simulink model "AnodeSubsystem_without_stack_Simplified"  (R2023a)
settings: Solver=VariableStepAuto  StartTime=0.0  StopTime=80  RelTol=1e-3
values from neighbouring files (symbols this model uses):
  anode_tube_D = 0.01    [Initialization_Anode.m]
  D = 0.01    [Initialization_Anode.m]
  densityHydrogen = 0.0899    [Initialization_Anode.m]
  Kv_VL6112 = 0.80    (= 0.8)    [Initialization_Anode.m]
  N2_T = [-56.55, -50:10:-10, -5:1:5, 10:10:350]    [Initialization_Anode.m]
  p_range = 0.005    [Initialization_Anode.m]
  r_max = 0.2    [Initialization_Anode.m]
  r_min = 1e-4    (= 0.0001)    [Initialization_Anode.m]
  responseTimeValve = 0.013    [Initialization_Anode.m]
libraries: fl_lib x64, nesl_utility x40, SimscapeFluids_lib x1
(part 2 of 2)

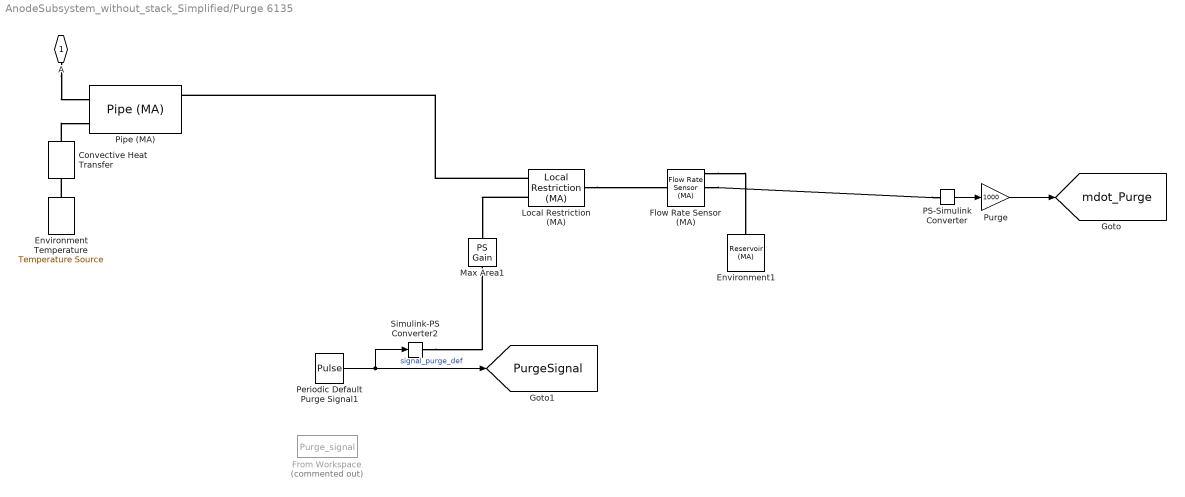
== system AnodeSubsystem_without_stack_Simplified/Purge 6135 ==
  Convective Heat Transfer : fl_lib/Thermal/Thermal Elements/Convective Heat Transfer  thermal_type=foundation.enum.constant_variable.constant  area=pi*anode_tube_D*1 m^2  heat_tr_coeff=20 W/(m^2 * K)  min_heat_tr_coeff=1e-3 W/(K*m^2)  T_specify=off  T_priority=None  T=0 K  T_nominal_specify=off  T_nominal_unit=K  T_nominal_value=1  Q_specify=off  Q_priority=None  Q=0 W  Q_nominal_specify=off  Q_nominal_unit=W  Q_nominal_value=1
  Environment Temperature : fl_lib/Thermal/Thermal Sources/Temperature Source  temperature=env_T degC
  Environment1 : fl_lib/Moist Air/Elements/Reservoir (MA)  pressure_spec=foundation.enum.pressure_spec.atmospheric  reservoir_pressure=0.101325 MPa  temperature_spec=foundation.enum.temperature_spec.atmospheric  reservoir_temperature=293.15 K  moisture_spec=foundation.enum.moistureSpec.RelativeHumidity  reservoir_RH=0.5  reservoir_x_w=0.01  reservoir_y_w=0.01  reservoir_HR=0.01  reservoir_Tw=287 K  trace_gas_spec=foundation.enum.trace_gas_spec.mass_fraction  reservoir_x_g=0.001  reservoir_y_g=0.001  RH_ws=1  area_A=0.01 m^2
  Flow Rate Sensor (MA) : fl_lib/Moist Air/Sensors/Flow Rate Sensor (MA)  mass_flow_measure=true  volumetric_flow_measure=false  volumetric_flow_conditions=foundation.enum.volumetric_flow_conditions.actual  p_std=0.101325 MPa  T_std=20 degC  RH_std=0.65  energy_flow_measure=true  vapor_flow_measure=false  gas_flow_measure=false
      settings: InternalSimscapePortConfiguration="{\"Bottom\":[{\"id\":\"PHI\",\"label\":\"φ\",\"type\":\"output\"}],\"Left\":[{\"id\":\"A\",\"label\":\"A\",\"type\":\"foundation.moist_air.moist_air\"}],\"Right\":[{\"id\":\"B\",\"label\":\"B\",\"type\":\"foundation.moist_air.moist_air\"},{\"id\":\"M\",\"label\":\"M\",\"type\":\"output\"}],\"Top\":[]}"
  From Workspace : FromWorkspace  Commented=on  VariableName=Purge_signal
  Local Restriction (MA) : fl_lib/Moist Air/Elements/Local Restriction (MA)  restriction_type=foundation.enum.restriction_type.variable  restriction_area=0.005 m^2  min_area=0.00001e-6 m^2  max_area=3.2e-6 m^2  area=0.00358 m^2  Cd=0.80  B_lam=0.999
      settings: LogSimulationData=on
  Max Area1 : fl_lib/Physical Signals/Functions/PS Gain  gain=3.2e-6 m^2
  PS-Simulink Converter : nesl_utility/PS-Simulink Converter  PhysicalDomain=network_engine_domain  SubClassName=ps_output  LeftPortType=input  RightPortType=output  PseudoPeriodic=off  Frequencies=[]  VectorFormat=inherit  Unit=inherit  AffineConversion=off
  Periodic Default Purge Signal1 : DiscretePulseGenerator  PulseType=Time based  Period=3  PulseWidth=5
  Pipe (MA) : fl_lib/Moist Air/Elements/Pipe (MA)  length=1 m  area=pi*anode_tube_D^2/4 m^2  Dh=anode_tube_D m  length_add=0.1 m  roughness=15e-6 m  Re_lam=2000  Re_tur=4000  shape_factor=64  Nu_lam=3.66  wall_condensation=simscape.enum.onoff.off  RH_ws=1  time_constant=1e-3 s  moisture_trace_gas_source=foundation.enum.moisture_trace_gas_source.none  moisture_source_spec=foundation.enum.moisture_source_spec.vapor  moisture_mass_flow=0 kg/s  moisture_temperature_spec=foundation.enum.temperature_spec.atmospheric  moisture_temperature=293.15 K  trace_gas_mass_flow=0 kg/s  trace_gas_temperature_spec=foundation.enum.temperature_spec.atmospheric  trace_gas_temperature=293.15 K  p_I_specify=on  p_I_priority=High  p_I=env_p MPa  p_I_nominal_specify=off  p_I_nominal_unit=MPa  p_I_nominal_value=1  T_I_specify=on  T_I_priority=High  T_I=env_T degC  T_I_nominal_specify=off  T_I_nominal_unit=K  T_I_nominal_value=1  RH_I_specify=off  RH_I_priority=High  RH_I=0  RH_I_nominal_specify=off  RH_I_nominal_unit=1  RH_I_nominal_value=1  x_w_I_specify=off  x_w_I_priority=None  x_w_I=0  x_w_I_nominal_specify=off  x_w_I_nominal_unit=1  x_w_I_nominal_value=1  y_w_I_specify=off  y_w_I_priority=None  y_w_I=0  y_w_I_nominal_specify=off  y_w_I_nominal_unit=1  y_w_I_nominal_value=1  HR_I_specify=off  HR_I_priority=None  HR_I=0  HR_I_nominal_specify=off  HR_I_nominal_unit=1  HR_I_nominal_value=1  x_g_I_specify=on  x_g_I_priority=None  x_g_I=0  x_g_I_nominal_specify=off  x_g_I_nominal_unit=1  x_g_I_nominal_value=1  y_g_I_specify=on  y_g_I_priority=High  y_g_I=tank_yH2  y_g_I_nominal_specify=off  y_g_I_nominal_unit=1  y_g_I_nominal_value=1
  Purge : Gain  Gain=1000
  Simulink-PS Converter2 : nesl_utility/Simulink-PS Converter  PhysicalDomain=network_engine_domain  SubClassName=ps_input  LeftPortType=input  RightPortType=output  PseudoPeriodic=off  Frequencies=[]  NoiseDistribution=none  NoiseParameters=[]  Unit=1  AffineConversion=off  FilteringAndDerivatives=provide  SimscapeFilterOrder=1  InputFilterTimeConstant=0.001  UdotUserProvided=0
  A : PMIOPort  Side=Left
  tag scope: PurgeSignal=global, mdot_Purge=global
  wires:
  PS-Simulink Converter/1 -> Purge/1
  Purge/1 -> [mdot_Purge]
  Periodic Default Purge Signal1/1 -> [PurgeSignal], Simulink-PS Converter2/1  "signal_purge_def"
  connections:
  Environment Temperature/LConn1 -- Convective Heat Transfer/RConn1
  Convective Heat Transfer/LConn1 -- Pipe (MA)/LConn2
  A/RConn1 -- Pipe (MA)/LConn1
  Local Restriction (MA)/LConn2 -- Max Area1/RConn1
  Simulink-PS Converter2/RConn1 -- Max Area1/LConn1
  Local Restriction (MA)/LConn1 -- Pipe (MA)/RConn1
  Local Restriction (MA)/RConn1 -- Flow Rate Sensor (MA)/LConn1
  Flow Rate Sensor (MA)/RConn1 -- Environment1/LConn1
  Flow Rate Sensor (MA)/RConn2 -- PS-Simulink Converter/LConn1

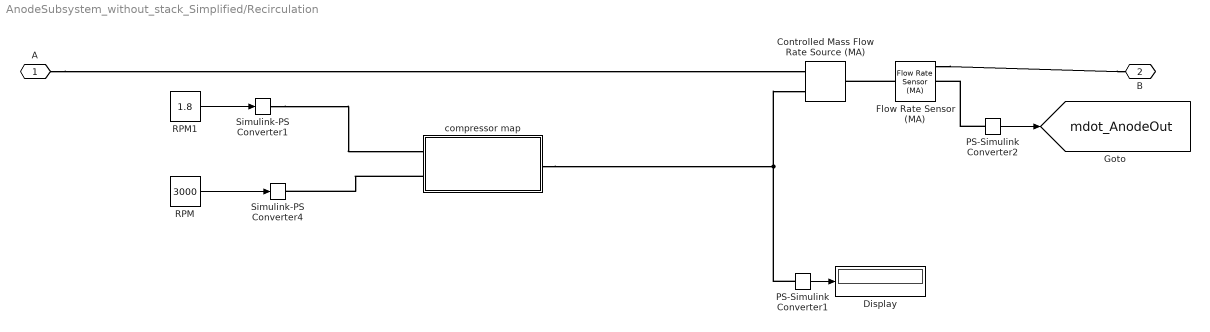
== system AnodeSubsystem_without_stack_Simplified/Recirculation ==
  Controlled Mass Flow Rate Source (MA) : fl_lib/Moist Air/Sources/Controlled Mass Flow Rate Source (MA)  power_spec=foundation.enum.power_spec.isentropic  area_A=pi*anode_tube_D^2/4 m^2  area_B=pi*anode_tube_D^2/4 m^2
      settings: InternalSimscapePortConfiguration="{\"Bottom\":[],\"Left\":[{\"id\":\"A\",\"label\":\"A\",\"type\":\"foundation.moist_air.moist_air\"},{\"id\":\"M\",\"label\":\"M\",\"type\":\"input\"}],\"Right\":[{\"id\":\"B\",\"label\":\"B\",\"type\":\"foundation.moist_air.moist_air\"}],\"Top\":[]}"
  Display : Display
  Flow Rate Sensor (MA) : fl_lib/Moist Air/Sensors/Flow Rate Sensor (MA)  mass_flow_measure=true  volumetric_flow_measure=false  volumetric_flow_conditions=foundation.enum.volumetric_flow_conditions.actual  p_std=0.101325 MPa  T_std=20 degC  RH_std=0.65  energy_flow_measure=true  vapor_flow_measure=false  gas_flow_measure=false
      settings: InternalSimscapePortConfiguration="{\"Bottom\":[{\"id\":\"PHI\",\"label\":\"φ\",\"type\":\"output\"}],\"Left\":[{\"id\":\"A\",\"label\":\"A\",\"type\":\"foundation.moist_air.moist_air\"}],\"Right\":[{\"id\":\"B\",\"label\":\"B\",\"type\":\"foundation.moist_air.moist_air\"},{\"id\":\"M\",\"label\":\"M\",\"type\":\"output\"}],\"Top\":[]}"
  PS-Simulink Converter1 : nesl_utility/PS-Simulink Converter  PhysicalDomain=network_engine_domain  SubClassName=ps_output  LeftPortType=input  RightPortType=output  PseudoPeriodic=off  Frequencies=[]  VectorFormat=inherit  Unit=inherit  AffineConversion=off
  PS-Simulink Converter2 : nesl_utility/PS-Simulink Converter  PhysicalDomain=network_engine_domain  SubClassName=ps_output  LeftPortType=input  RightPortType=output  PseudoPeriodic=off  Frequencies=[]  VectorFormat=inherit  Unit=inherit  AffineConversion=off
  RPM : Constant  Value=3000
  RPM1 : Constant  Value=1.8
  Simulink-PS Converter1 : nesl_utility/Simulink-PS Converter  PhysicalDomain=network_engine_domain  SubClassName=ps_input  LeftPortType=input  RightPortType=output  PseudoPeriodic=off  Frequencies=[]  NoiseDistribution=none  NoiseParameters=[]  Unit=1  AffineConversion=off  FilteringAndDerivatives=provide  SimscapeFilterOrder=1  InputFilterTimeConstant=0.001  UdotUserProvided=0
  Simulink-PS Converter4 : nesl_utility/Simulink-PS Converter  PhysicalDomain=network_engine_domain  SubClassName=ps_input  LeftPortType=input  RightPortType=output  PseudoPeriodic=off  Frequencies=[]  NoiseDistribution=none  NoiseParameters=[]  Unit=1  AffineConversion=off  FilteringAndDerivatives=provide  SimscapeFilterOrder=1  InputFilterTimeConstant=0.001  UdotUserProvided=0
  compressor map : Subsystem
  A : PMIOPort  Side=Left
  B : PMIOPort  Port=2  Side=Right
  tag scope: mdot_AnodeOut=global
  wires:
  RPM/1 -> Simulink-PS Converter4/1
  PS-Simulink Converter1/1 -> Display/1
  PS-Simulink Converter2/1 -> [mdot_AnodeOut]
  RPM1/1 -> Simulink-PS Converter1/1
  connections:
  A/RConn1 -- Controlled Mass Flow Rate Source (MA)/LConn1
  compressor map/LConn2 -- Simulink-PS Converter4/RConn1
  compressor map/RConn1 -- PS-Simulink Converter1/LConn1 -- Controlled Mass Flow Rate Source (MA)/LConn2
  Flow Rate Sensor (MA)/LConn1 -- Controlled Mass Flow Rate Source (MA)/RConn1
  Flow Rate Sensor (MA)/RConn1 -- B/RConn1
  PS-Simulink Converter2/LConn1 -- Flow Rate Sensor (MA)/RConn2
  Simulink-PS Converter1/RConn1 -- compressor map/LConn1

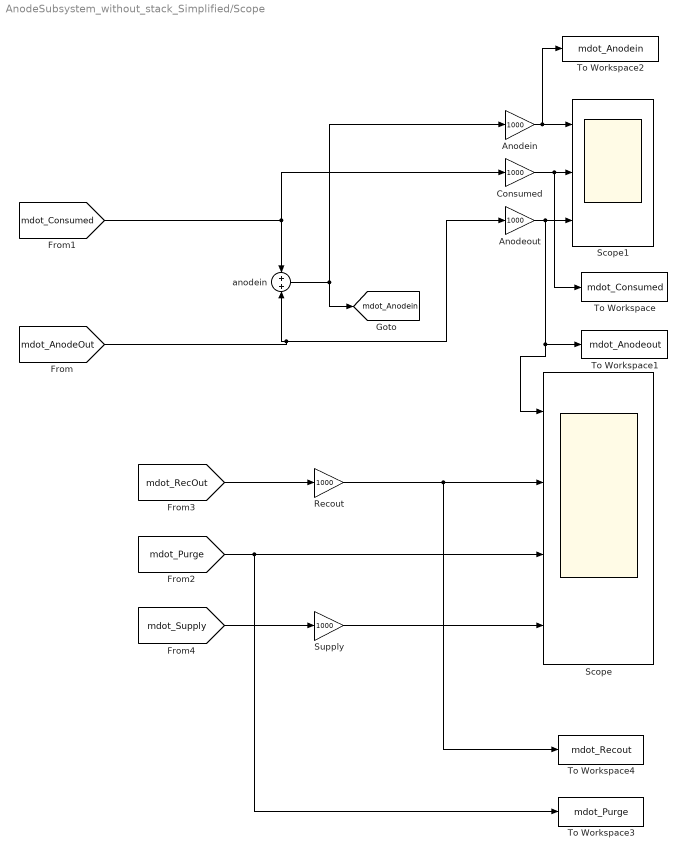
== system AnodeSubsystem_without_stack_Simplified/Scope ==
  Anodein : Gain  Gain=1000
  Anodeout : Gain  Gain=1000
  Consumed : Gain  Gain=1000
  Recout : Gain  Gain=1000
  Scope : Scope  NumInputPorts=4
  Scope1 : Scope  NumInputPorts=3
  Supply : Gain  Gain=1000
  To Workspace : ToWorkspace  VariableName=mdot_Consumed  SaveFormat=Structure With Time  SampleTime=-1
  To Workspace1 : ToWorkspace  VariableName=mdot_Anodeout  SaveFormat=Structure With Time  SampleTime=-1
  To Workspace2 : ToWorkspace  VariableName=mdot_Anodein  SaveFormat=Structure With Time  SampleTime=-1
  To Workspace3 : ToWorkspace  VariableName=mdot_Purge  SaveFormat=Structure With Time  SampleTime=-1
  To Workspace4 : ToWorkspace  VariableName=mdot_Recout  SaveFormat=Structure With Time  SampleTime=-1
  anodein : Sum
  tag scope: mdot_Anodein=global
  wires:
  [mdot_Consumed] -> anodein/1, Consumed/1
  [mdot_AnodeOut] -> Anodeout/1, anodein/2
  Anodein/1 -> To Workspace2/1, Scope1/1
  Anodeout/1 -> Scope/1, To Workspace1/1, Scope1/3
  Consumed/1 -> To Workspace/1, Scope1/2
  [mdot_Purge] -> To Workspace3/1, Scope/3
  anodein/1 -> [mdot_Anodein], Anodein/1
  Recout/1 -> To Workspace4/1, Scope/2
  [mdot_RecOut] -> Recout/1
  [mdot_Supply] -> Supply/1
  Supply/1 -> Scope/4

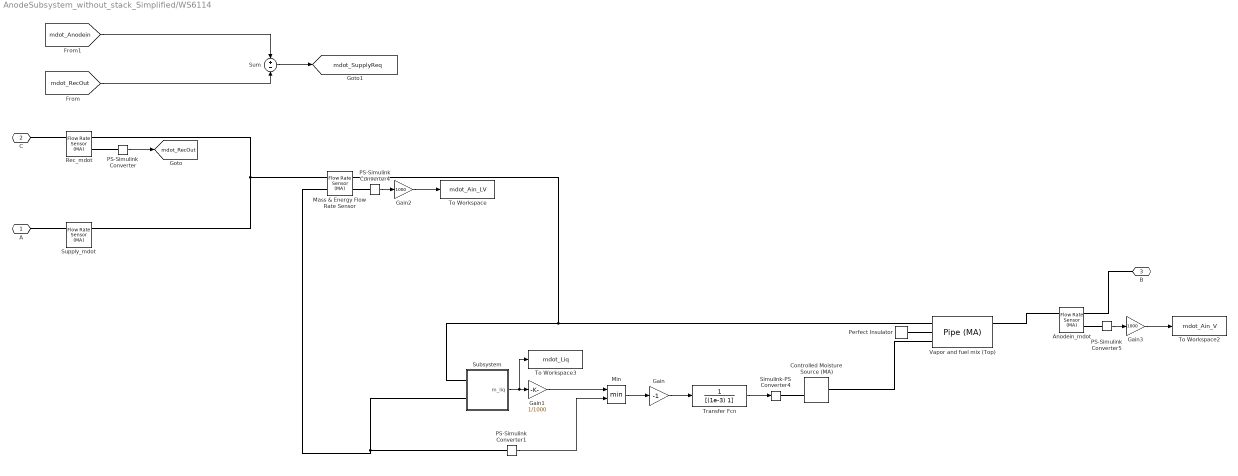
== system AnodeSubsystem_without_stack_Simplified/WS6114 ==
  Anodein_mdot : fl_lib/Moist Air/Sensors/Flow Rate Sensor (MA)  mass_flow_measure=true  volumetric_flow_measure=false  volumetric_flow_conditions=foundation.enum.volumetric_flow_conditions.actual  p_std=0.101325 MPa  T_std=20 degC  RH_std=0.65  energy_flow_measure=false  vapor_flow_measure=true  gas_flow_measure=false
      settings: InternalSimscapePortConfiguration="{\"Bottom\":[],\"Left\":[{\"id\":\"A\",\"label\":\"A\",\"type\":\"foundation.moist_air.moist_air\"},{\"id\":\"Mw\",\"label\":\"Mw\",\"type\":\"output\"}],\"Right\":[{\"id\":\"B\",\"label\":\"B\",\"type\":\"foundation.moist_air.moist_air\"},{\"id\":\"M\",\"label\":\"M\",\"type\":\"output\"}],\"Top\":[]}"
  Controlled Moisture Source (MA) : fl_lib/Moist Air/Sources/Moisture & Trace Gas Sources/Controlled Moisture Source (MA)  moisture_source_spec=foundation.enum.moisture_source_spec.liquid  Phi_S_specify=off  Phi_S_priority=None  Phi_S=0 kW  Phi_S_nominal_specify=off  Phi_S_nominal_unit=kW  Phi_S_nominal_value=1  mdot_w_S_specify=off  mdot_w_S_priority=None  mdot_w_S=0 kg/s  mdot_w_S_nominal_specify=off  mdot_w_S_nominal_unit=kg/s  mdot_w_S_nominal_value=1
      settings: InternalSimscapePortConfiguration="{\"Bottom\":[],\"Left\":[{\"id\":\"S\",\"label\":\"S\",\"type\":\"foundation.moist_air.moist_air_source\"}],\"Right\":[{\"id\":\"M\",\"label\":\"M\",\"type\":\"input\"},{\"id\":\"T\",\"label\":\"T\",\"type\":\"input\"}],\"Top\":[]}"
  Gain : Gain  Gain=-1
  Gain1 : Gain  Gain=1/1000
  Gain2 : Gain  Gain=1000
  Gain3 : Gain  Gain=1000
  "Mass & Energy Flow Rate Sensor " : fl_lib/Moist Air/Sensors/Flow Rate Sensor (MA)  mass_flow_measure=true  volumetric_flow_measure=false  volumetric_flow_conditions=foundation.enum.volumetric_flow_conditions.actual  p_std=0.101325 MPa  T_std=20 degC  RH_std=0.65  energy_flow_measure=false  vapor_flow_measure=true  gas_flow_measure=false
      settings: InternalSimscapePortConfiguration="{\"Bottom\":[],\"Left\":[{\"id\":\"A\",\"label\":\"A\",\"type\":\"foundation.moist_air.moist_air\"},{\"id\":\"Mw\",\"label\":\"Mw\",\"type\":\"output\"}],\"Right\":[{\"id\":\"B\",\"label\":\"B\",\"type\":\"foundation.moist_air.moist_air\"},{\"id\":\"M\",\"label\":\"M\",\"type\":\"output\"}],\"Top\":[]}"
  Min : MinMax  Inputs=2
  PS-Simulink Converter{,1,4..5} (4 alike) : nesl_utility/PS-Simulink Converter  PhysicalDomain=network_engine_domain  SubClassName=ps_output  LeftPortType=input  RightPortType=output  PseudoPeriodic=off  Frequencies=[]  VectorFormat=inherit  Unit=inherit  AffineConversion=off
  Perfect Insulator : fl_lib/Thermal/Thermal Elements/Perfect Insulator  T_specify=off  T_priority=None  T=0 K  T_nominal_specify=off  T_nominal_unit=K  T_nominal_value=1
  Rec_mdot : fl_lib/Moist Air/Sensors/Flow Rate Sensor (MA)  mass_flow_measure=true  volumetric_flow_measure=false  volumetric_flow_conditions=foundation.enum.volumetric_flow_conditions.actual  p_std=0.101325 MPa  T_std=20 degC  RH_std=0.65  energy_flow_measure=false  vapor_flow_measure=true  gas_flow_measure=false
      settings: InternalSimscapePortConfiguration="{\"Bottom\":[],\"Left\":[{\"id\":\"A\",\"label\":\"A\",\"type\":\"foundation.moist_air.moist_air\"},{\"id\":\"Mw\",\"label\":\"Mw\",\"type\":\"output\"}],\"Right\":[{\"id\":\"B\",\"label\":\"B\",\"type\":\"foundation.moist_air.moist_air\"},{\"id\":\"M\",\"label\":\"M\",\"type\":\"output\"}],\"Top\":[]}"
  Simulink-PS Converter4 : nesl_utility/Simulink-PS Converter  PhysicalDomain=network_engine_domain  SubClassName=ps_input  LeftPortType=input  RightPortType=output  PseudoPeriodic=off  Frequencies=[]  NoiseDistribution=none  NoiseParameters=[]  Unit=1  AffineConversion=off  FilteringAndDerivatives=provide  SimscapeFilterOrder=1  InputFilterTimeConstant=0.001  UdotUserProvided=0
  Subsystem : Subsystem
  Sum : Sum  Inputs=+-
  Supply_mdot : fl_lib/Moist Air/Sensors/Flow Rate Sensor (MA)  mass_flow_measure=true  volumetric_flow_measure=false  volumetric_flow_conditions=foundation.enum.volumetric_flow_conditions.actual  p_std=0.101325 MPa  T_std=20 degC  RH_std=0.65  energy_flow_measure=false  vapor_flow_measure=true  gas_flow_measure=false
      settings: InternalSimscapePortConfiguration="{\"Bottom\":[],\"Left\":[{\"id\":\"A\",\"label\":\"A\",\"type\":\"foundation.moist_air.moist_air\"},{\"id\":\"Mw\",\"label\":\"Mw\",\"type\":\"output\"}],\"Right\":[{\"id\":\"B\",\"label\":\"B\",\"type\":\"foundation.moist_air.moist_air\"},{\"id\":\"M\",\"label\":\"M\",\"type\":\"output\"}],\"Top\":[]}"
  To Workspace : ToWorkspace  VariableName=mdot_Ain_LV  SaveFormat=Structure With Time  SampleTime=-1
  To Workspace2 : ToWorkspace  VariableName=mdot_Ain_V  SaveFormat=Structure With Time  SampleTime=-1
  To Workspace3 : ToWorkspace  VariableName=mdot_Liq  SaveFormat=Structure With Time  SampleTime=-1
  Transfer Fcn : TransferFcn  Denominator=[(1e-3) 1]
  Vapor and fuel mix (Top) : fl_lib/Moist Air/Elements/Pipe (MA)  length=0.25 m  area=pi*0.05^2/4 m^2  Dh=0.05 m  length_add=0.1 m  roughness=15e-6 m  Re_lam=2000  Re_tur=4000  shape_factor=64  Nu_lam=3.66  wall_condensation=simscape.enum.onoff.off  RH_ws=1  time_constant=1e-3 s  moisture_trace_gas_source=foundation.enum.moisture_trace_gas_source.controlled  moisture_source_spec=foundation.enum.moisture_source_spec.vapor  moisture_mass_flow=0 kg/s  moisture_temperature_spec=foundation.enum.temperature_spec.atmospheric  moisture_temperature=293.15 K  trace_gas_mass_flow=0 kg/s  trace_gas_temperature_spec=foundation.enum.temperature_spec.atmospheric  trace_gas_temperature=293.15 K  p_I_specify=on  p_I_priority=High  p_I=env_p MPa  p_I_nominal_specify=off  p_I_nominal_unit=MPa  p_I_nominal_value=1  T_I_specify=on  T_I_priority=High  T_I=env_T degC  T_I_nominal_specify=off  T_I_nominal_unit=K  T_I_nominal_value=1  RH_I_specify=off  RH_I_priority=High  RH_I=0  RH_I_nominal_specify=off  RH_I_nominal_unit=1  RH_I_nominal_value=1  x_w_I_specify=off  x_w_I_priority=None  x_w_I=0  x_w_I_nominal_specify=off  x_w_I_nominal_unit=1  x_w_I_nominal_value=1  y_w_I_specify=off  y_w_I_priority=None  y_w_I=0  y_w_I_nominal_specify=off  y_w_I_nominal_unit=1  y_w_I_nominal_value=1  HR_I_specify=off  HR_I_priority=None  HR_I=0  HR_I_nominal_specify=off  HR_I_nominal_unit=1  HR_I_nominal_value=1  x_g_I_specify=on  x_g_I_priority=None  x_g_I=0  x_g_I_nominal_specify=off  x_g_I_nominal_unit=1  x_g_I_nominal_value=1  y_g_I_specify=on  y_g_I_priority=High  y_g_I=tank_yH2  y_g_I_nominal_specify=off  y_g_I_nominal_unit=1  y_g_I_nominal_value=1
      settings: InternalSimscapePortConfiguration="{\"Bottom\":[],\"Left\":[{\"id\":\"A\",\"label\":\"A\",\"type\":\"foundation.moist_air.moist_air\"},{\"id\":\"H\",\"label\":\"H\",\"type\":\"foundation.thermal.thermal\"},{\"id\":\"S\",\"label\":\"S\",\"type\":\"foundation.moist_air.moist_air_source\"}],\"Right\":[{\"id\":\"B\",\"label\":\"B\",\"type\":\"foundation.moist_air.moist_air\"},{\"id\":\"W\",\"label\":\"W\",\"type\":\"output\"},{\"id\":\"F\",\"label\":\"F\",\"type\":\"output\"}],\"Top\":[]}"
  A : PMIOPort  Side=Left
  C : PMIOPort  Port=2  Side=Left
  B : PMIOPort  Port=3  Side=Right
  tag scope: mdot_RecOut=global, mdot_SupplyReq=global
  wires:
  PS-Simulink Converter1/1 -> Min/2
  Subsystem/1(m_liq) -> To Workspace3/1, Gain1/1
  Transfer Fcn/1 -> Simulink-PS Converter4/1
  Min/1 -> Gain/1
  Gain/1 -> Transfer Fcn/1
  Gain1/1 -> Min/1
  PS-Simulink Converter/1 -> [mdot_RecOut]
  [mdot_RecOut] -> Sum/2
  [mdot_Anodein] -> Sum/1
  Sum/1 -> [mdot_SupplyReq]
  Gain2/1 -> To Workspace/1
  PS-Simulink Converter4/1 -> Gain2/1
  Gain3/1 -> To Workspace2/1
  PS-Simulink Converter5/1 -> Gain3/1
  connections:
  C/RConn1 -- Rec_mdot/LConn1
  Supply_mdot/LConn1 -- A/RConn1
  Rec_mdot/RConn1 -- Supply_mdot/RConn1 -- "Mass & Energy Flow Rate Sensor "/LConn1
  "Mass & Energy Flow Rate Sensor "/RConn1 -- Subsystem/LConn1 -- Vapor and fuel mix (Top)/LConn1
  Subsystem/LConn2 -- "Mass & Energy Flow Rate Sensor "/LConn2 -- PS-Simulink Converter1/LConn1
  Controlled Moisture Source (MA)/LConn1 -- Vapor and fuel mix (Top)/LConn3
  Simulink-PS Converter4/RConn1 -- Controlled Moisture Source (MA)/RConn1
  Perfect Insulator/LConn1 -- Vapor and fuel mix (Top)/LConn2
  Anodein_mdot/RConn1 -- B/RConn1
  Anodein_mdot/LConn1 -- Vapor and fuel mix (Top)/RConn1
  PS-Simulink Converter/LConn1 -- Rec_mdot/RConn2
  PS-Simulink Converter5/LConn1 -- Anodein_mdot/RConn2
  PS-Simulink Converter4/LConn1 -- "Mass & Energy Flow Rate Sensor "/RConn2

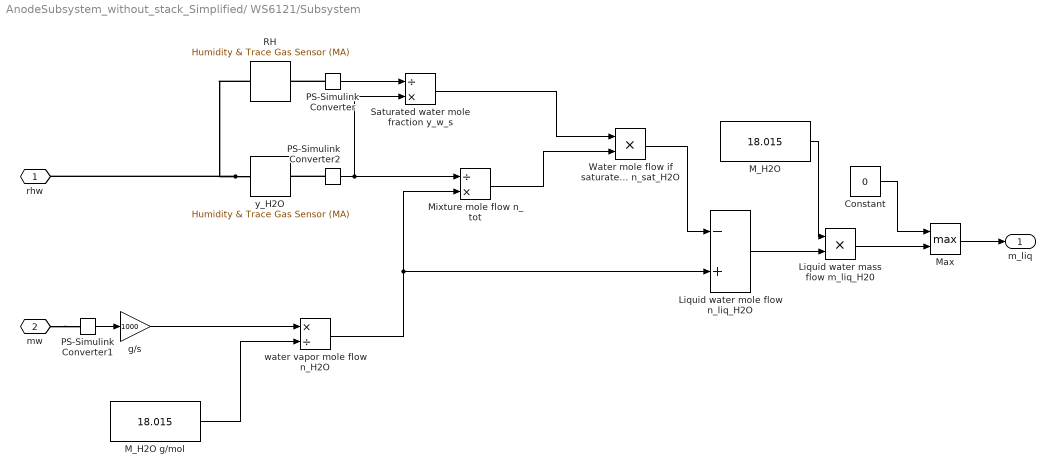
== system AnodeSubsystem_without_stack_Simplified/ WS6121/Subsystem ==
  Constant : Constant  Value=0
  Liquid water mass flow m_liq_H20 : Product
  Liquid water mole flow n_liq_H2O : Sum  Inputs=-+
  M_H2O : Constant  Value=18.015
  M_H2O g/mol : Constant  Value=18.015
  Max : MinMax  Function=max  Inputs=2
  Mixture mole flow n_tot : Product  Inputs=/*
  PS-Simulink Converter : nesl_utility/PS-Simulink Converter  PhysicalDomain=network_engine_domain  SubClassName=ps_output  LeftPortType=input  RightPortType=output  PseudoPeriodic=off  Frequencies=[]  VectorFormat=inherit  Unit=inherit  AffineConversion=off
  PS-Simulink Converter1 : nesl_utility/PS-Simulink Converter  PhysicalDomain=network_engine_domain  SubClassName=ps_output  LeftPortType=input  RightPortType=output  PseudoPeriodic=off  Frequencies=[]  VectorFormat=inherit  Unit=inherit  AffineConversion=off
  PS-Simulink Converter2 : nesl_utility/PS-Simulink Converter  PhysicalDomain=network_engine_domain  SubClassName=ps_output  LeftPortType=input  RightPortType=output  PseudoPeriodic=off  Frequencies=[]  VectorFormat=inherit  Unit=inherit  AffineConversion=off
  RH : fl_lib/Moist Air/Sensors/Humidity & Trace Gas Sensor (MA)  moisture_on=true  moisture_spec=foundation.enum.moistureSpec.RelativeHumidity  trace_gas_on=false  trace_gas_spec=foundation.enum.trace_gas_spec.mole_fraction
      settings: InternalSimscapePortConfiguration="{\"Bottom\":[],\"Left\":[{\"id\":\"A\",\"label\":\"A\",\"type\":\"foundation.moist_air.moist_air\"}],\"Right\":[{\"id\":\"W\",\"label\":\"W\",\"type\":\"output\"}],\"Top\":[]}"
  Saturated water mole fraction y_w_s : Product  Inputs=/*
  Water mole flow if saturated n_sat_H2O : Product
  g/s : Gain  Gain=1000
  water vapor mole flow n_H2O : Product  Inputs=*/
  y_H2O : fl_lib/Moist Air/Sensors/Humidity & Trace Gas Sensor (MA)  moisture_on=true  moisture_spec=foundation.enum.moistureSpec.MoleFraction  trace_gas_on=false  trace_gas_spec=foundation.enum.trace_gas_spec.mole_fraction
      settings: InternalSimscapePortConfiguration="{\"Bottom\":[],\"Left\":[{\"id\":\"A\",\"label\":\"A\",\"type\":\"foundation.moist_air.moist_air\"}],\"Right\":[{\"id\":\"W\",\"label\":\"W\",\"type\":\"output\"}],\"Top\":[]}"
  rhw : PMIOPort  Side=Left
  mw : PMIOPort  Port=2  Side=Left
  m_liq : Outport
  wires:
  Constant/1 -> Max/1
  Max/1 -> m_liq/1
  water vapor mole flow n_H2O/1 -> Mixture mole flow n_tot/2, Liquid water mole flow n_liq_H2O/2
  PS-Simulink Converter1/1 -> g/s/1
  Liquid water mole flow n_liq_H2O/1 -> Liquid water mass flow m_liq_H20/2
  PS-Simulink Converter/1 -> Saturated water mole fraction y_w_s/1
  Liquid water mass flow m_liq_H20/1 -> Max/2
  Water mole flow if saturated n_sat_H2O/1 -> Liquid water mole flow n_liq_H2O/1
  g/s/1 -> water vapor mole flow n_H2O/1
  Saturated water mole fraction y_w_s/1 -> Water mole flow if saturated n_sat_H2O/1
  PS-Simulink Converter2/1 -> Mixture mole flow n_tot/1, Saturated water mole fraction y_w_s/2
  Mixture mole flow n_tot/1 -> Water mole flow if saturated n_sat_H2O/2
  M_H2O/1 -> Liquid water mass flow m_liq_H20/1
  M_H2O g/mol/1 -> water vapor mole flow n_H2O/2
  connections:
  y_H2O/LConn1 -- rhw/RConn1 -- RH/LConn1
  PS-Simulink Converter2/LConn1 -- y_H2O/RConn1
  PS-Simulink Converter/LConn1 -- RH/RConn1
  mw/RConn1 -- PS-Simulink Converter1/LConn1

== system AnodeSubsystem_without_stack_Simplified/ WS6121/ValveControl ==
  Simulink-PS Converter1 : nesl_utility/Simulink-PS Converter  PhysicalDomain=network_engine_domain  SubClassName=ps_input  LeftPortType=input  RightPortType=output  PseudoPeriodic=off  Frequencies=[]  NoiseDistribution=none  NoiseParameters=[]  Unit=m^2  AffineConversion=off  FilteringAndDerivatives=provide  SimscapeFilterOrder=1  InputFilterTimeConstant=0.001  UdotUserProvided=0
  Step2 : Step  Time=10  SampleTime=0
  Transfer Fcn2 : TransferFcn  Numerator=[4.75e-6]  Denominator=[1 1]
  Cmd : PMIOPort  Side=Right
  wires:
  Transfer Fcn2/1 -> Simulink-PS Converter1/1
  Step2/1 -> Transfer Fcn2/1
  connections:
  Simulink-PS Converter1/RConn1 -- Cmd/RConn1

== system AnodeSubsystem_without_stack_Simplified/APRV VL6112/Valve Command Controller ==
  note: Valve Lift Command Controller calculates valvelift signal for an
      | ideal controller, to reach desired vave outlet pressure, assuming
      | a linear relation between valve lift and Kvs.
      | (funcionality validated 09.05.2023)
  Control Inlet Pressure [bar] : Inport
  Control Inlet Temperature [K] : Inport  Port=2
  Desired Control Outlet Pressure [bar] : Inport  Port=3
  Control Outlet Mass Flow Rate [g/s] : Inport  Port=4
  Display : Display
  Kv [m^3/h] : Constant  Value=Kv_VL6112
  Saturation : Saturate  UpperLimit=1  LowerLimit=0
  Scope : Scope  NumInputPorts=2
  Standard Density [kg/(m^3)] : Constant  Value=densityHydrogen
  Valve Lift Command Control : MATLAB Function  TreatAsAtomicUnit=on
  Valve Lift Signal [-] : Outport
  wires:
  Desired Control Outlet Pressure [bar]/1 -> Valve Lift Command Control/3(p2)  "p_valve_out_desired"
  Control Inlet Pressure [bar]/1 -> Valve Lift Command Control/2(p1)  "p_valve_in"
  Control Outlet Mass Flow Rate [g/s]/1 -> Valve Lift Command Control/1(m_dot), Scope/1  "m_dot_valve"
  Control Inlet Temperature [K]/1 -> Valve Lift Command Control/4(T1)  "T_valve_in"
  Kv [m^3/h]/1 -> Valve Lift Command Control/5(Kvs)
  Standard Density [kg/(m^3)]/1 -> Valve Lift Command Control/6(rho_std)
  Valve Lift Command Control/1(lift_signal) -> Saturation/1
  Saturation/1 -> Scope/2, Valve Lift Signal [-]/1  "lift_signal_command"
  Valve Lift Command Control/2(W) -> Display/1

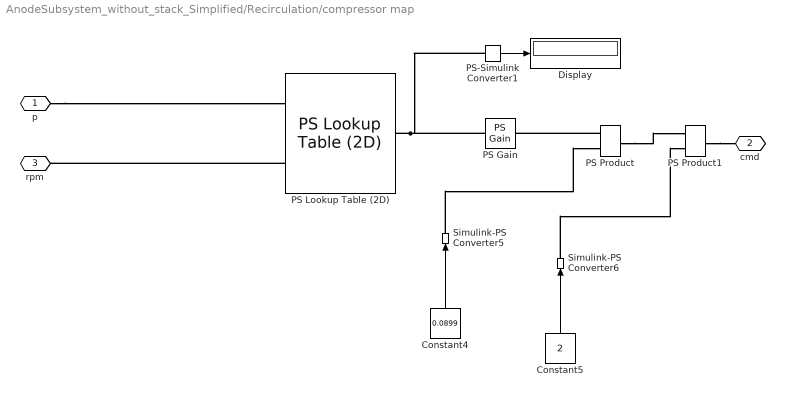
== system AnodeSubsystem_without_stack_Simplified/Recirculation/compressor map ==
  Constant4 : Constant  Value=0.0899
  Constant5 : Constant  Value=2
  Display : Display
  PS Gain : fl_lib/Physical Signals/Functions/PS Gain  gain=1/3600
  PS Lookup Table (2D) : fl_lib/Physical Signals/Lookup Tables/PS Lookup Table (2D)  x1=comp6122_p_out  x2=comp6122_rpm  f=comp6122_V_dot  interp_method=simscape.enum.interpolation.linear  extrap_method=simscape.enum.extrapolation.linear
  PS Product : fl_lib/Physical Signals/Functions/PS Product
  PS Product1 : fl_lib/Physical Signals/Functions/PS Product
  PS-Simulink Converter1 : nesl_utility/PS-Simulink Converter  PhysicalDomain=network_engine_domain  SubClassName=ps_output  LeftPortType=input  RightPortType=output  PseudoPeriodic=off  Frequencies=[]  VectorFormat=inherit  Unit=inherit  AffineConversion=off
  Simulink-PS Converter5 : nesl_utility/Simulink-PS Converter  PhysicalDomain=network_engine_domain  SubClassName=ps_input  LeftPortType=input  RightPortType=output  PseudoPeriodic=off  Frequencies=[]  NoiseDistribution=none  NoiseParameters=[]  Unit=1  AffineConversion=on  FilteringAndDerivatives=provide  SimscapeFilterOrder=1  InputFilterTimeConstant=0.001  UdotUserProvided=0
  Simulink-PS Converter6 : nesl_utility/Simulink-PS Converter  PhysicalDomain=network_engine_domain  SubClassName=ps_input  LeftPortType=input  RightPortType=output  PseudoPeriodic=off  Frequencies=[]  NoiseDistribution=none  NoiseParameters=[]  Unit=1  AffineConversion=on  FilteringAndDerivatives=provide  SimscapeFilterOrder=1  InputFilterTimeConstant=0.001  UdotUserProvided=0
  p : PMIOPort  Side=Left
  cmd : PMIOPort  Port=2  Side=Right
  rpm : PMIOPort  Port=3  Side=Left
  wires:
  Constant4/1 -> Simulink-PS Converter5/1
  Constant5/1 -> Simulink-PS Converter6/1
  PS-Simulink Converter1/1 -> Display/1
  connections:
  Simulink-PS Converter5/RConn1 -- PS Product/LConn2
  PS Lookup Table (2D)/RConn1 -- PS Gain/LConn1 -- PS-Simulink Converter1/LConn1
  PS Product/RConn1 -- PS Product1/LConn1
  PS Product/LConn1 -- PS Gain/RConn1
  PS Lookup Table (2D)/LConn2 -- rpm/RConn1
  Simulink-PS Converter6/RConn1 -- PS Product1/LConn2
  PS Product1/RConn1 -- cmd/RConn1
  p/RConn1 -- PS Lookup Table (2D)/LConn1

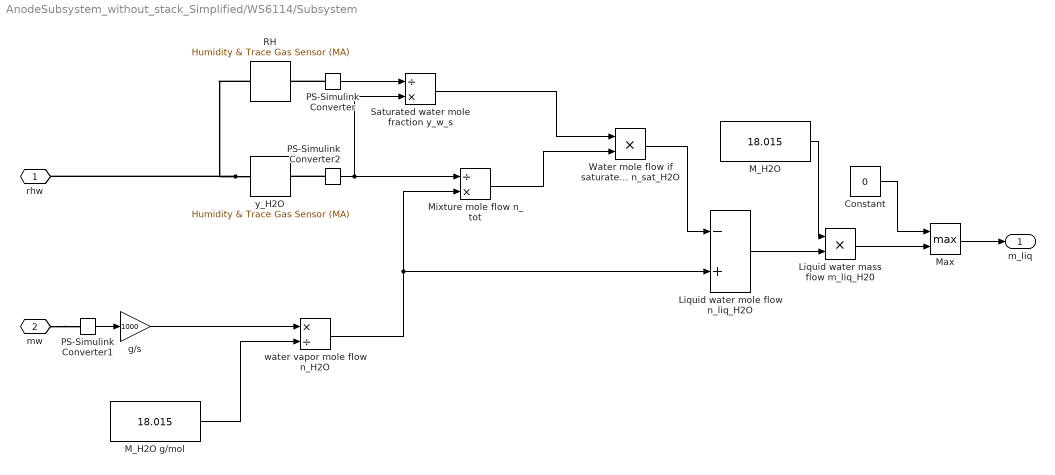
== system AnodeSubsystem_without_stack_Simplified/WS6114/Subsystem ==
  Constant : Constant  Value=0
  Liquid water mass flow m_liq_H20 : Product
  Liquid water mole flow n_liq_H2O : Sum  Inputs=-+
  M_H2O : Constant  Value=18.015
  M_H2O g/mol : Constant  Value=18.015
  Max : MinMax  Function=max  Inputs=2
  Mixture mole flow n_tot : Product  Inputs=/*
  PS-Simulink Converter : nesl_utility/PS-Simulink Converter  PhysicalDomain=network_engine_domain  SubClassName=ps_output  LeftPortType=input  RightPortType=output  PseudoPeriodic=off  Frequencies=[]  VectorFormat=inherit  Unit=inherit  AffineConversion=off
  PS-Simulink Converter1 : nesl_utility/PS-Simulink Converter  PhysicalDomain=network_engine_domain  SubClassName=ps_output  LeftPortType=input  RightPortType=output  PseudoPeriodic=off  Frequencies=[]  VectorFormat=inherit  Unit=inherit  AffineConversion=off
  PS-Simulink Converter2 : nesl_utility/PS-Simulink Converter  PhysicalDomain=network_engine_domain  SubClassName=ps_output  LeftPortType=input  RightPortType=output  PseudoPeriodic=off  Frequencies=[]  VectorFormat=inherit  Unit=inherit  AffineConversion=off
  RH : fl_lib/Moist Air/Sensors/Humidity & Trace Gas Sensor (MA)  moisture_on=true  moisture_spec=foundation.enum.moistureSpec.RelativeHumidity  trace_gas_on=false  trace_gas_spec=foundation.enum.trace_gas_spec.mole_fraction
      settings: InternalSimscapePortConfiguration="{\"Bottom\":[],\"Left\":[{\"id\":\"A\",\"label\":\"A\",\"type\":\"foundation.moist_air.moist_air\"}],\"Right\":[{\"id\":\"W\",\"label\":\"W\",\"type\":\"output\"}],\"Top\":[]}"
  Saturated water mole fraction y_w_s : Product  Inputs=/*
  Water mole flow if saturated n_sat_H2O : Product
  g/s : Gain  Gain=1000
  water vapor mole flow n_H2O : Product  Inputs=*/
  y_H2O : fl_lib/Moist Air/Sensors/Humidity & Trace Gas Sensor (MA)  moisture_on=true  moisture_spec=foundation.enum.moistureSpec.MoleFraction  trace_gas_on=false  trace_gas_spec=foundation.enum.trace_gas_spec.mole_fraction
      settings: InternalSimscapePortConfiguration="{\"Bottom\":[],\"Left\":[{\"id\":\"A\",\"label\":\"A\",\"type\":\"foundation.moist_air.moist_air\"}],\"Right\":[{\"id\":\"W\",\"label\":\"W\",\"type\":\"output\"}],\"Top\":[]}"
  rhw : PMIOPort  Side=Left
  mw : PMIOPort  Port=2  Side=Left
  m_liq : Outport
  wires:
  Constant/1 -> Max/1
  Max/1 -> m_liq/1
  water vapor mole flow n_H2O/1 -> Mixture mole flow n_tot/2, Liquid water mole flow n_liq_H2O/2
  PS-Simulink Converter1/1 -> g/s/1
  Liquid water mole flow n_liq_H2O/1 -> Liquid water mass flow m_liq_H20/2
  PS-Simulink Converter/1 -> Saturated water mole fraction y_w_s/1
  Liquid water mass flow m_liq_H20/1 -> Max/2
  Water mole flow if saturated n_sat_H2O/1 -> Liquid water mole flow n_liq_H2O/1
  g/s/1 -> water vapor mole flow n_H2O/1
  Saturated water mole fraction y_w_s/1 -> Water mole flow if saturated n_sat_H2O/1
  PS-Simulink Converter2/1 -> Mixture mole flow n_tot/1, Saturated water mole fraction y_w_s/2
  Mixture mole flow n_tot/1 -> Water mole flow if saturated n_sat_H2O/2
  M_H2O/1 -> Liquid water mass flow m_liq_H20/1
  M_H2O g/mol/1 -> water vapor mole flow n_H2O/2
  connections:
  y_H2O/LConn1 -- rhw/RConn1 -- RH/LConn1
  PS-Simulink Converter2/LConn1 -- y_H2O/RConn1
  PS-Simulink Converter/LConn1 -- RH/RConn1
  mw/RConn1 -- PS-Simulink Converter1/LConn1

== matlab function AnodeSubsystem_without_stack_Simplified/APRV VL6112/Valve Command Controller/Valve Lift Command Control ==
  data: m_dot input; p1 input; p2 input; T1 input; Kvs input; lift_signal output; rho_std input; W output
function [lift_signal,W]  = fcn(m_dot,p1,p2,T1,Kvs,rho_std)

% calculation based on Bürkert. Direktwirkendes 2-Wege-Standard-Proportionalventil. Datenblatt
% for calculation based on Swagelok. Valve Sizing. Technical Bulletin:
% check calculation_valve_formulas_comparison

% determine optimum valve opening based on pressure ratio for subscritical conditions
% Kvs - valve coefficient [m^3/h] at fully valve open
% lift_signal = Kv/Kvs (linear assumption)

dp = max(0,p1 - p2);            % avoid complex square root

% distinction of flow characteristics based on pressure drop
if p2/p1 > 0.5
    % low pressure drop - subsonic flow
    lift_signal = m_dot*3.6/(Kvs*514)*sqrt(T1/(p2*dp*rho_std));
    W=1;
  
else 
    % high pressure drop - sonic flow (independent of downstream pressure)
    %lift_signal = 0.05;
    lift_signal = m_dot*3.6/(Kvs*257*p1)*sqrt(T1/rho_std);
     W=2;
end
